simulink model "project"  (R2021a)
settings: Solver=VariableStepAuto  StartTime=0.0  StopTime=70  RelTol=1e-3
undefined symbols (not defined in the file): Down, Up
libraries: spsCurrentMeasurementLib x5, spsVoltageMeasurementLib x3, spsMeanLib x2, spsDCMachineLib x1, spsDCVoltageSourceLib x1, spsDiodeLib x1, spsIdealSwitchLib x1, eePwmGenerator x1, eePowerMeasurement x1, spsSeriesRLCBranchLib x1, spsThreePhaseSourceLib x1, spsUniversalBridgeLib x1
settings Model: Creator=akara  LastModifiedBy=akara

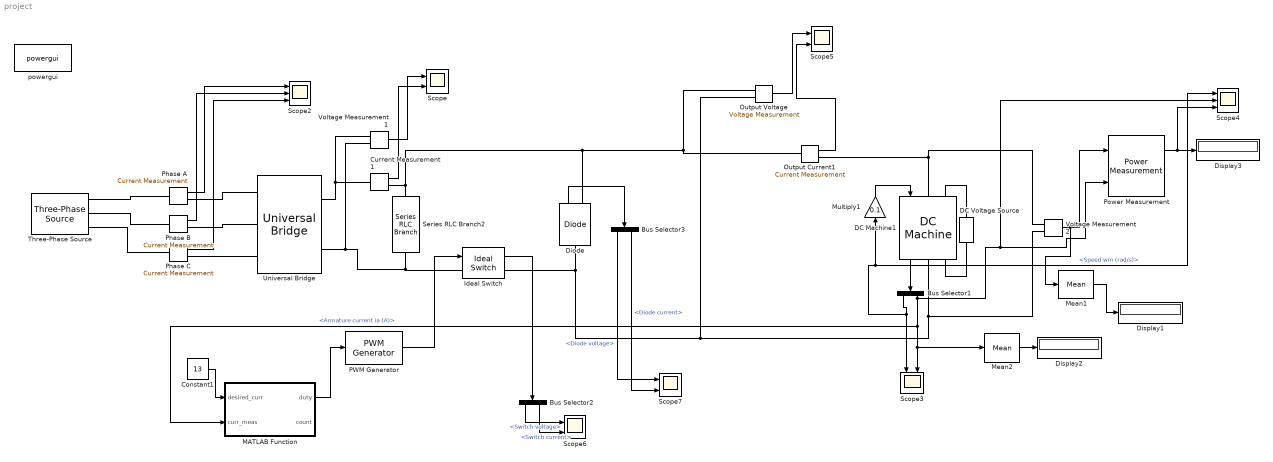
== system project ==
  Bus Selector1 : BusSelector  OutputSignals=Speed wm (rad/s),Armature current ia (A)
  Bus Selector2 : BusSelector  OutputSignals=Switch voltage,Switch current
  Bus Selector3 : BusSelector  OutputSignals=Diode voltage,Diode current
  Constant1 : Constant  Value=13
  Current Measurement1 : spsCurrentMeasurementLib/Current Measurement  PhasorSimulation=off  OutputType=Complex  PSBequivalent=0
  DC Machine1 : spsDCMachineLib/DC Machine  PresetModel=No  MechanicalLoad=Torque TL  FieldType=Wound  ShowDetailedParameters=on  MeasurementBus=off  RLa=[0.8 12.5e-3]  RLf="[ 240  120]"  Laf=1.8  MachineConstant=Torque constant (N.m/A)  Ke=1.8  Kt=1.8  J=1  Bm=0  Tf=0  w0=0  Ifinit=0.625  TsPowergui=0  TsBlock=-1
  DC Voltage Source : spsDCVoltageSourceLib/DC Voltage Source  Amplitude=150  Measurements=None
  Diode : spsDiodeLib/Diode  Ron=0.001  Lon=0  Vf=0.8  IC=0  UseSnubber=0  Rs=500  Cs=250e-9  Measurements=on
  Display1 : Display
  Display2 : Display
  Display3 : Display
  Ideal Switch : spsIdealSwitchLib/Ideal Switch  Ron=0.001  Lon=0  IC=0  Rs=1e5  Cs=inf  Measurements=on
  MATLAB Function : MATLAB Function  TreatAsAtomicUnit=on
  Mean1 : spsMeanLib/Mean  Freq=60  Vinit=0  Ts=0
  Mean2 : spsMeanLib/Mean  Freq=60  Vinit=0  Ts=0
  Multiply1 : Gain  Gain=0.1
  Output Current1 : spsCurrentMeasurementLib/Current Measurement  PhasorSimulation=off  OutputType=Complex  PSBequivalent=0
  Output Voltage : spsVoltageMeasurementLib/Voltage Measurement  PhasorSimulation=off  OutputType=Complex  PSBequivalent=0
  PWM Generator : eePwmGenerator/PWM Generator  CarrCount=Up-Down  Tper=2e-4  Ts=0
  Phase A : spsCurrentMeasurementLib/Current Measurement  PhasorSimulation=off  OutputType=Complex  PSBequivalent=0
  Phase B : spsCurrentMeasurementLib/Current Measurement  PhasorSimulation=off  OutputType=Complex  PSBequivalent=0
  Phase C : spsCurrentMeasurementLib/Current Measurement  PhasorSimulation=off  OutputType=Complex  PSBequivalent=0
  Power Measurement : eePowerMeasurement/Power Measurement  LabelModeActiveChoice=Continuous  F=60  K=[0 1 2 3]  Ts=0
      settings: SourceProductBaseCode=PS
  Scope{,3,5..7} (5 alike) : Scope  NumInputPorts=2
  Scope2 : Scope  NumInputPorts=3
  Scope4 : Scope  NumInputPorts=3
  Series RLC Branch2 : spsSeriesRLCBranchLib/Series RLC Branch  LConnTagsString=__new0  RConnTagsString=__new0  BranchType=C  Resistance=1  Inductance=1e-3  SetiL0=off  InitialCurrent=0  Capacitance=440e-6  Setx0=off  InitialVoltage=0  Measurements=None
  Three-Phase Source : spsThreePhaseSourceLib/Three-Phase Source  InternalConnection=Yg  VoltagePhases=off  Voltage=160  PhaseAngle=0  Voltage_phases=[25e3 25e3 25e3]/sqrt(3)  PhaseAngles_phases=[0 -120 +120]  Frequency=50  NonIdealSource=on  SpecifyImpedance=off  Resistance=0  Inductance=0  ShortCircuitLevel=100e6  BaseVoltage=180  XRratio=7  BusType=swing  Pref=10e3  Qref=0  Prefabc=[10e3, 10e3, 10e3]  Qrefabc=[0, 0, 0]  Qmin=-inf  Qmax=inf
  Universal Bridge : spsUniversalBridgeLib/Universal Bridge  Arms=3  SnubberResistance=1e5  SnubberCapacitance=inf  Device=Diodes  Ron=1e-3  Lon=0  ForwardVoltages="[  0  0  ]"  ForwardVoltage=0  GTOparameters=[ 10e-6 , 20e-6 ]  IGBTparameters=[ 1e-6 , 2e-6 ]  Measurements=None  Measurements_2=None  converterType=Rectifier
  Voltage Measurement1 : spsVoltageMeasurementLib/Voltage Measurement  PhasorSimulation=off  OutputType=Complex  PSBequivalent=0
  Voltage Measurement2 : spsVoltageMeasurementLib/Voltage Measurement  PhasorSimulation=off  OutputType=Complex  PSBequivalent=0
  powergui : spspowerguiLib/powergui  Priority=1  SimulationMode=Continuous  SampleTime=1e-5  frequency=60  Iterations=50  frequencyindice=50  Pbase=100e6  ErrMax=1e-4  UnitsV=kV  UnitsW=MW  buscounter=0  FunctionMessages=off  echomessages=off  EnableUseOfTLC=off  CurrentSourceSwitches=off  DisableSnubberDevices=off  DisableRonSwitches=off  DisableVfSwitches=off  DisplayEquations=off  AutomaticDiscreteSolvers=off  SolverType=Tustin/Backward Euler (TBE)  Interpol=off  ExternalGateDelay=off  methode=off  Ts=100  x0status=blocks  SPID=on  SwTol=0  HookPort=off  NonlinearTolerance=1e-4  nMaxIteration=100  ContinueOnMaxIteration=off  RestoreLinks=warning  ResistiveCurrentMeasurement=off  Frange=[0:2:500]  Ylog=off  Xlog=on  ShowGrid=off  save=off  variable=ZData  structure=0  ZoomFFT=off  StartTime=0.0  cycles=1  DisplayStyle=1  fundamental=60  FreqAxis=off  MaxFrequency=1000  frequencyindicesteady=1  RmsSteady=1  display=off
  wires:
  Voltage Measurement1/1 -> Scope/1
  Current Measurement1/1 -> Scope/2
  Power Measurement/1 -> Scope4/3, Display3/1
  Mean2/1 -> Display2/1
  Mean1/1 -> Display1/1
  DC Machine1/1 -> Bus Selector1/1
  Voltage Measurement2/1 -> Power Measurement/1, Mean1/1
  Bus Selector1/2 -> Scope4/2, Power Measurement/2, MATLAB Function/2(curr_meas), Scope3/2, Mean2/1  "<Armature current ia (A)>"
  PWM Generator/1 -> Ideal Switch/1
  Output Voltage/1 -> Scope5/1
  Constant1/1 -> MATLAB Function/1(desired_curr)
  MATLAB Function/1(duty) -> PWM Generator/1
  Phase A/1 -> Scope2/1
  Phase B/1 -> Scope2/2
  Phase C/1 -> Scope2/3
  Output Current1/1 -> Scope5/2
  Bus Selector1/1 -> Multiply1/1, Scope4/1, Scope3/1  "<Speed wm (rad/s)>"
  Multiply1/1 -> DC Machine1/1
  Ideal Switch/1 -> Bus Selector2/1
  Bus Selector2/2 -> Scope6/2  "<Switch current>"
  Bus Selector2/1 -> Scope6/1  "<Switch voltage>"
  Diode/1 -> Bus Selector3/1
  Bus Selector3/1 -> Scope7/1  "<Diode voltage>"
  Bus Selector3/2 -> Scope7/2  "<Diode current>"
  connections:
  Voltage Measurement1/LConn1 -- Universal Bridge/RConn1 -- Current Measurement1/LConn1
  Series RLC Branch2/RConn1 -- Ideal Switch/LConn1 -- Voltage Measurement1/LConn2 -- Universal Bridge/RConn2
  Ideal Switch/RConn1 -- Output Voltage/LConn2 -- DC Machine1/RConn1 -- Voltage Measurement2/LConn2 -- Diode/LConn1
  Current Measurement1/RConn1 -- Output Voltage/LConn1 -- Output Current1/LConn1 -- Diode/RConn1 -- Series RLC Branch2/LConn1
  DC Machine1/RConn2 -- DC Voltage Source/LConn1
  DC Machine1/LConn2 -- DC Voltage Source/RConn1
  Three-Phase Source/RConn1 -- Phase A/LConn1
  Three-Phase Source/RConn2 -- Phase B/LConn1
  Three-Phase Source/RConn3 -- Phase C/LConn1
  Phase A/RConn1 -- Universal Bridge/LConn1
  Phase B/RConn1 -- Universal Bridge/LConn2
  Phase C/RConn1 -- Universal Bridge/LConn3
  Voltage Measurement2/LConn1 -- Output Current1/RConn1 -- DC Machine1/LConn1

== matlab function project/MATLAB Function ==
  settings: updateMethod=DISCRETE  sampleTime=10e-6
  data: desired_curr input; duty output; curr_meas input; count output
function [duty, count]= fcn(desired_curr, curr_meas)
persistent tick
persistent calcduty
persistent integral
if(isempty(tick))
    tick=0;
end
if(isempty(calcduty))
    calcduty=0;
end
if(isempty(integral))
    integral=-0.5;
end

if(tick == 0)
    integral = integral + (desired_curr-curr_meas)/10;
    if(integral<-0.6)
        integral = -0.6;
    elseif(integral>0.6)
        integral = 0.6;
    end
    calcduty = (desired_curr-curr_meas)*0.5+integral;
    if(desired_curr>curr_meas)
        calcduty = calcduty+0.0001;
    elseif(desired_curr<curr_meas)
        calcduty = calcduty-0.0001;
    end
end
tick = tick + 1;

if(tick==10) 
    tick = 0;
end

if(calcduty>1)
    calcduty = 1;
elseif(calcduty<0)
    calcduty=0;
end
count = tick;
duty = calcduty;
end
